simulink model "Modelo_Red_Mitigación_final"  (R2019b)
settings: Solver=VariableStepAuto  StartTime=0.0  StopTime=2.5  RelTol=1e-3
InitFcn:
  | Ts=20e-6;
undefined symbols (not defined in the file): D1, Delta, Ion, Lithium
libraries: powerlib x371, powerlib_meascontrol x286, simulink x50, simulink_extras x20, electricdrivelib x16
(part 4 of 11)

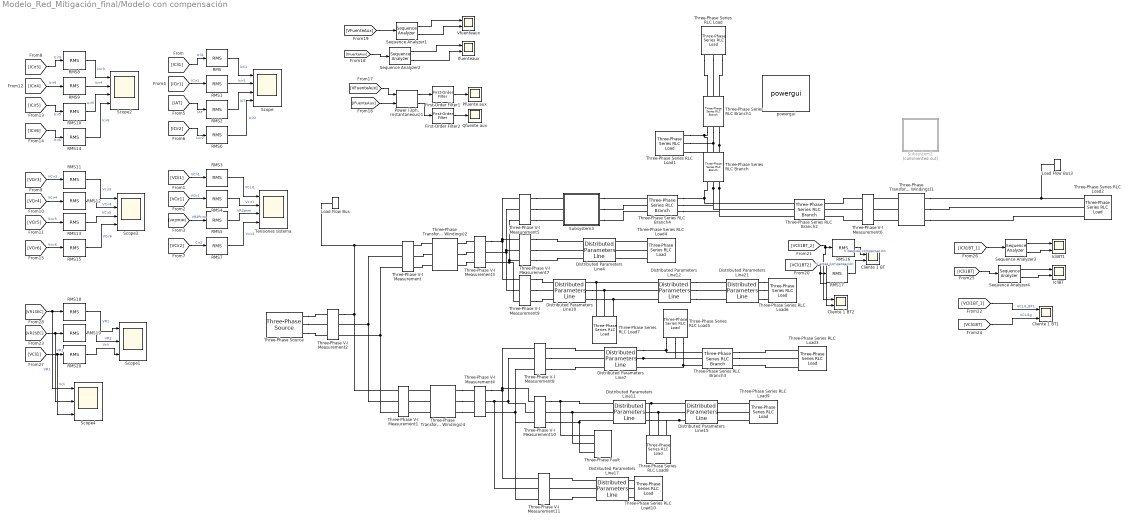
== system Modelo_Red_Mitigación_final/Modelo con compensación ==
  Cliente 1 BT : Scope  NumInputPorts=2
  Cliente 1 BT1 : Scope  NumInputPorts=3
  Cliente 1 BT2 : Scope  NumInputPorts=2
  Distributed Parameters Line10 : powerlib/Elements/Distributed Parameters Line  Phases=3  Frequency=60  Resistance=[0.213 0.639]  Inductance=[0.78e-3 2.35e-3]  Capacitance=[15e-9 15e-9]  Length=3  x1=[-2e-05 3.60953176170516e-09 32175.0070560431 -19325.0634978567;-1e-05 3.60559101207762e-09 32247.6320174573 -19203.6295402532]  x2=[-2e-05 3.3920787146718e-09 31687.8811035473 -19346.7961292865;-1e-05 3.38863307732371e-09 31760.5914564267 -19227.1984344751]  x3=[-2e-05 -6.04879747397163e-11 -137.471205101226 265.134927538772;-1e-05 -6.06175334127226e-11 -138.469760977244 264.614790455632]  x4=[-2e-05 7.88128095264096e-11 416.613031958925 -434.907199032997;-1e-05 7.89310008588255e-11 418.249629092382 -433.333518127575]  x5=1.78115131305569e-05  V1=ones(3,3)  V2=ones(3,3)  I1=ones(3,3)  I2=ones(3,3)  nHarmo=1  Measurements=None
      settings: SourceProductName=Simscape Electrical
  Distributed Parameters Line11 : powerlib/Elements/Distributed Parameters Line  Phases=3  Frequency=60  Resistance=[0.269 0.807]  Inductance=[0.85e-3 2.56e-3]  Capacitance=[15e-9 15e-9]  Length=18  x1=[-0.00012 2.25515335002305e-09 31483.0427639054 -20454.4474545806;-0.00011 2.26415722602629e-09 31559.9303096165 -20335.6141091991;-0.0001 2.27312892334362e-09 31636.3693188597 -20216.4917497281;-9e-05 2.28206831446736e-09 31712.3587052676 -20097.0820691601;-8e-05 2.29097527234899e-09 31787.8973888629 -19977.3867645708;-7e-05 2.29984967040091e-09 31862.9842960736 -19857.4075370956;-6e-05 2.30869138249829e-09 31937.6183597485 -19737.1460919048;-5e-05 2.31750028298082e-09 32011.7985191725 -19616.6041381797;-4e-05 2.32627624665453e-09 32085.5237200813 -19495.7833890884;-3e-05 2.33501914879354e-09 32158.7929146765 -19374.6855617611;-2e-05 2.34372886514188e-09 32231.6050616407 -19253.312377266;-1e-05 2.35240527191519e-09 32303.9591261522 -19131.6655605847]  x2=[-0.00012 1.94941502653526e-09 29675.6367944921 -20128.6580942059;-0.00011 1.95749754273358e-09 29751.3089897787 -20016.6408077573;-0.0001 1.9655522385589e-09 29826.5583531098 -19904.3390405358;-9e-05 1.97357899953614e-09 29901.3838150256 -19791.7543885982;-8e-05 1.98157771158727e-09 29975.7843120904 -19678.8884520216;-7e-05 1.98954826103289e-09 30049.7587869086 -19565.7428348808;-6e-05 1.99749053459384e-09 30123.3061881392 -19452.3191452254;-5e-05 2.00540441939284e-09 30196.4254705107 -19338.6189950572;-4e-05 2.01328980295607e-09 30269.1155948363 -19224.6440003069;-3e-05 2.02114657321477e-09 30341.3755280285 -19110.3957808115;-2e-05 2.02897461850684e-09 30413.2042431137 -18995.8759602911;-1e-05 2.03677382757844e-09 30484.6007192467 -18881.0861663258]  x3=[-0.00012 5.15773485528783e-12 9.28421720699589 123.310848994962;-0.00011 5.11579108823116e-12 8.81928138472589 123.344973326285;-0.0001 5.0737746144593e-12 8.35422022094588 123.377344652512;-9e-05 5.03168603111934e-12 7.88904032520442 123.407962513576;-8e-05 4.98952593638322e-12 7.42374830873751 123.436826474328;-7e-05 4.9472949294392e-12 6.95835078437463 123.463936124547;-6e-05 4.90499361048336e-12 6.49285436644475 123.489291078947;-5e-05 4.86262258071109e-12 6.02726567068236 123.512890977175;-4e-05 4.82018244230851e-12 5.5615913141334 123.534735483827;-3e-05 4.77767379844393e-12 5.09583791506126 123.554824288443;-2e-05 4.73509725325926e-12 4.63001209285268 123.573157105516;-1e-05 4.69245341186146e-12 4.16412046792371 123.589733674497]  x4=[-0.00012 5.1467508786483e-12 241.702417431134 -294.296225052516;-0.00011 5.23026920454686e-12 242.810167870273 -293.382939263731;-0.0001 5.31371319674279e-12 243.914467439464 -292.465483853974;-9e-05 5.39708166931226e-12 245.015300444167 -291.543871862318;-8e-05 5.48037343740475e-12 246.112651239108 -290.618116386908;-7e-05 5.56358731725985e-12 247.206504228504 -289.68823058478;-6e-05 5.64672212622414e-12 248.296843866281 -288.754227671669;-5e-05 5.72977668276798e-12 249.383654656301 -287.816120921824;-4e-05 5.81274980650226e-12 250.466921152576 -286.873923667818;-3e-05 5.89564031819523e-12 251.546627959491 -285.92764930036;-2e-05 5.97844703978925e-12 252.622759732024 -284.977311268103;-1e-05 6.06116879441752e-12 253.695301175959 -284.022923077453]  x5=0.000111541920370774  V1=ones(3,3)  V2=ones(3,3)  I1=ones(3,3)  I2=ones(3,3)  nHarmo=1  Measurements=None
      settings: SourceProductName=Simscape Electrical
  Distributed Parameters Line12 : powerlib/Elements/Distributed Parameters Line  Phases=3  Frequency=60  Resistance=[0.269 0.807]  Inductance=[0.85e-3 2.56e-3]  Capacitance=[15e-9 15e-9]  Length=6  x1=[-4e-05 3.40065095400314e-09 0 0;-3e-05 3.39730015910595e-09 31614.7203957361 -19466.1188633006;-2e-05 3.39390108105356e-09 31687.8811035473 -19346.7961292865;-1e-05 3.39045376815439e-09 31760.5914564267 -19227.1984344751]  x2=[-4e-05 3.45797591228592e-09 0 0;-3e-05 3.45530178649685e-09 30837.5027565935 -19380.3404703211;-2e-05 3.45257855322106e-09 30910.3456112392 -19263.9483803875;-1e-05 3.44980625116172e-09 30982.7491614535 -19147.2825071065]  x3=[-4e-05 -3.69816611276407e-12 0 0;-3e-05 -3.61783769618688e-12 -40.501984824249 176.337783353379;-2e-05 -3.53745786212792e-12 -41.1664732198401 176.183841754365;-1e-05 -3.45702775296255e-12 -41.8303765487246 176.027396192976]  x4=[-4e-05 1.96504684539837e-11 0 0;-3e-05 1.95629170007581e-11 300.866672819785 -339.753955836259;-2e-05 1.94750875151792e-11 302.145374033175 -338.617303560211;-1e-05 1.93869812454986e-11 303.419781092 -337.475838782748]  x5=3.71806401235912e-05  V1=ones(3,3)  V2=ones(3,3)  I1=ones(3,3)  I2=ones(3,3)  nHarmo=1  Measurements=None
      settings: SourceProductName=Simscape Electrical
  Distributed Parameters Line15 : powerlib/Elements/Distributed Parameters Line  Phases=3  Frequency=60  Resistance=[0.269 0.807]  Inductance=[0.85e-3 2.56e-3]  Capacitance=[15e-9 15e-9]  Length=12  x1=[-8e-05 1.98156914110105e-09 0 0;-7e-05 1.98954076159097e-09 0 0;-6e-05 1.99748410630282e-09 0 0;-5e-05 2.00539906234407e-09 30196.4254705107 -19338.6189950572;-4e-05 2.01328551722569e-09 30269.1155948363 -19224.6440003069;-3e-05 2.02114335886368e-09 30341.3755280285 -19110.3957808115;-2e-05 2.02897247558074e-09 30413.2042431137 -18995.8759602911;-1e-05 2.03677275610778e-09 30484.6007192467 -18881.0861663258]  x2=[-8e-05 1.91667238330513e-09 0 0;-7e-05 1.92456740683708e-09 0 0;-6e-05 1.93243507800613e-09 0 0;-5e-05 1.94027528499527e-09 29816.1536069817 -19273.9878791696;-4e-05 1.94808791637781e-09 29888.6027805703 -19161.4469314506;-3e-05 1.95587286111894e-09 29960.6271709548 -19048.6336571567;-2e-05 1.96363000857739e-09 30032.2257545092 -18935.5496596142;-1e-05 1.97135924850691e-09 30103.3975136591 -18822.1965459972]  x3=[-8e-05 2.70938359599311e-12 0 0;-7e-05 2.71078492729944e-12 0 0;-6e-05 2.71214773235161e-12 0 0;-5e-05 2.71347199178116e-12 86.3403246372415 -15.5892894445469;-4e-05 2.71475768676741e-12 86.3984811911008 -15.2636840808873;-3e-05 2.71600479903781e-12 86.455409831299 -14.9378617864907;-2e-05 2.71721331086812e-12 86.5111097487539 -14.611827192013;-1e-05 2.71838320508272e-12 86.5655801518465 -14.2855849311276]  x4=[-8e-05 6.06852121097726e-12 0 0;-7e-05 6.10206473358783e-12 0 0;-6e-05 6.13552153235158e-12 0 0;-5e-05 6.16889113177335e-12 161.91207626267 -146.998141908763;-4e-05 6.20217305759727e-12 162.465094324763 -146.38670462294;-3e-05 6.23536683681349e-12 163.015803398247 -145.773186858016;-2e-05 6.26847199766495e-12 163.564195656329 -145.157597333438;-1e-05 6.30148806965402e-12 164.11026330514 -144.539944798094]  x5=7.43612802471824e-05  V1=ones(3,3)  V2=ones(3,3)  I1=ones(3,3)  I2=ones(3,3)  nHarmo=1  Measurements=None
      settings: SourceProductName=Simscape Electrical
  Distributed Parameters Line17 : powerlib/Elements/Distributed Parameters Line  Phases=3  Frequency=60  Resistance=[0.213 0.639]  Inductance=[0.78e-3 2.35e-3]  Capacitance=[15e-9 15e-9]  Length=18  x1=[-0.00011 2.26415722602629e-09 31559.9303096165 -20335.6141091991;-0.0001 2.27312892334362e-09 31636.3693188597 -20216.4917497281;-9e-05 2.28206831446736e-09 31712.3587052676 -20097.0820691601;-8e-05 2.29097527234899e-09 31787.8973888629 -19977.3867645708;-7e-05 2.29984967040091e-09 31862.9842960736 -19857.4075370956;-6e-05 2.30869138249829e-09 31937.6183597485 -19737.1460919048;-5e-05 2.31750028298082e-09 32011.7985191725 -19616.6041381797;-4e-05 2.32627624665453e-09 32085.5237200813 -19495.7833890884;-3e-05 2.33501914879354e-09 32158.7929146765 -19374.6855617611;-2e-05 2.34372886514188e-09 32231.6050616407 -19253.312377266;-1e-05 2.35240527191519e-09 32303.9591261522 -19131.6655605847]  x2=[-0.00011 2.16599636455895e-09 30839.7793585705 -20381.2716559546;-0.0001 2.17462439466361e-09 30916.3956097717 -20264.8638707302;-9e-05 2.18322151854208e-09 30992.5724705577 -20148.1680769337;-8e-05 2.1917876140102e-09 31068.3088582867 -20031.1859330708;-7e-05 2.20032255932479e-09 31143.6036965769 -19913.9191017167;-6e-05 2.20882623318538e-09 31218.4559153221 -19796.3692494926;-5e-05 2.21729851473596e-09 31292.8644507065 -19678.538047042;-4e-05 2.22573928356664e-09 31366.8282452201 -19560.4271690073;-3e-05 2.23414841971541e-09 31440.3462476737 -19442.0382940054;-2e-05 2.24252580366984e-09 31513.4174132138 -19323.3731046042;-1e-05 2.25087131636876e-09 31586.0407033373 -19204.4332872989]  x3=[-0.00011 5.75160708206705e-12 65.9317893508161 -5.21472769211793;-0.0001 5.74612435792413e-12 65.9509798461658 -4.96613423438911;-9e-05 5.74055996863501e-12 65.9692330321091 -4.71747019690026;-8e-05 5.73491399328197e-12 65.9865486492278 -4.46873911371776;-7e-05 5.72918651210683e-12 66.0029264514285 -4.21994451986088;-6e-05 5.72337760650976e-12 66.0183662059466 -3.97108995125151;-5e-05 5.71748735904818e-12 66.0328676933488 -3.7221789446639;-4e-05 5.71151585343554e-12 66.0464307075371 -3.47321503767442;-3e-05 5.70546317454015e-12 66.0590550557509 -3.22420176861127;-2e-05 5.69932940838398e-12 66.0707405585703 -2.97514267650421;-1e-05 5.69311464214142e-12 66.0814870499183 -2.72604130103422]  x4=[-0.00011 4.31568373195511e-12 202.227351702517 -174.253957712798;-0.0001 4.36167015875297e-12 202.882835041406 -173.490342096467;-9e-05 4.40759459656329e-12 203.535434966127 -172.724260798352;-8e-05 4.45345639269816e-12 204.185142201791 -171.955724706166;-7e-05 4.49925489535994e-12 204.831947514619 -171.184744742506;-6e-05 4.54498945365053e-12 205.475841712076 -170.411331864706;-5e-05 4.59065941758063e-12 206.116815643 -169.635497064673;-4e-05 4.63626413807896e-12 206.754860197734 -168.857251368738;-3e-05 4.68180296700149e-12 207.389966308251 -168.076605837494;-2e-05 4.72727525714066e-12 208.022124948288 -167.293571565643;-1e-05 4.77268036223458e-12 208.651327133471 -166.508159681835]  x5=0.000106869078783341  V1=ones(3,3)  V2=ones(3,3)  I1=ones(3,3)  I2=ones(3,3)  nHarmo=1  Measurements=None
      settings: SourceProductName=Simscape Electrical
  Distributed Parameters Line21 : powerlib/Elements/Distributed Parameters Line  Phases=3  Frequency=60  Resistance=[0.269 0.807]  Inductance=[0.85e-3 2.56e-3]  Capacitance=[15e-9 15e-9]  Length=3  x1=[-2e-05 3.45441977735251e-09 30910.3456112392 -19263.9483803875;-1e-05 3.45163637093425e-09 30982.7491614535 -19147.2825071065]  x2=[-2e-05 3.12977626724445e-09 30521.2143171991 -19221.4149453172;-1e-05 3.12742225506452e-09 30593.4602857292 -19106.216361226]  x3=[-2e-05 -7.08035851296492e-11 -43.7280619986038 177.821448028224;-1e-05 -7.09955174729478e-11 -44.398120740149 177.655333890518]  x4=[-2e-05 8.23431902033655e-11 300.811121285787 -339.602032284616;-1e-05 8.25181278003377e-11 302.089250156992 -338.465590512005]  x5=1.85903200617956e-05  V1=ones(3,3)  V2=ones(3,3)  I1=ones(3,3)  I2=ones(3,3)  nHarmo=1  Measurements=None
      settings: SourceProductName=Simscape Electrical
  Distributed Parameters Line4 : powerlib/Elements/Distributed Parameters Line  Phases=3  Frequency=60  Resistance=[0.213 0.639]  Inductance=[0.78e-3 2.35e-3]  Capacitance=[15e-9 15e-9]  Length=9  x1=[-6e-05 3.62494578097809e-09 31879.9448486981 -19808.035609231;-5e-05 3.62118313403904e-09 31954.3926645073 -19687.7105752568;-4e-05 3.61736902207213e-09 32028.3863376657 -19567.1057353365;-3e-05 3.61350349928436e-09 32101.9248165591 -19446.2228035317;-2e-05 3.60958662061336e-09 32175.0070560431 -19325.0634978567;-1e-05 3.60561844172663e-09 32247.6320174573 -19203.6295402532]  x2=[-6e-05 3.32131517644419e-09 31220.7541322128 -19854.186340228;-5e-05 3.3181246812965e-09 31295.3806160466 -19736.34606287;-4e-05 3.3148870282524e-09 31369.5623232492 -19618.225288348;-3e-05 3.31160226332611e-09 31443.2981995346 -19499.8256954195;-2e-05 3.30827043320141e-09 31516.5871969527 -19381.148966805;-1e-05 3.30489158523098e-09 31589.4282739045 -19262.1967891634]  x3=[-6e-05 -2.09677278907869e-11 9.19435123996087 67.3100361697703;-5e-05 -2.10349486785391e-11 8.940533646812 67.3442196629359;-4e-05 -2.11018705131096e-11 8.6865889888901 67.3774460456733;-3e-05 -2.1168492443391e-11 8.43252087531085 67.4097148457621;-2e-05 -2.12348135225382e-11 8.17833291694453 67.4410256045912;-1e-05 -2.13008328079819e-11 7.92402872636468 67.4713778771654]  x4=[-6e-05 3.87950361892921e-11 264.77686067222 -241.746580654783;-5e-05 3.88437674883829e-11 265.686340119013 -240.746679893785;-4e-05 3.88919467315569e-11 266.592043574815 -239.743357589571;-3e-05 3.89395732340802e-11 267.493958167574 -238.736628001573;-2e-05 3.8986646319075e-11 268.392071079089 -237.726505437646;-1e-05 3.90331653175284e-11 269.286369545186 -236.713004253869]  x5=5.34345393916706e-05  V1=ones(3,3)  V2=ones(3,3)  I1=ones(3,3)  I2=ones(3,3)  nHarmo=1  Measurements=None
      settings: SourceProductName=Simscape Electrical
  Distributed Parameters Line7 : powerlib/Elements/Distributed Parameters Line  Phases=3  Frequency=60  Resistance=[0.213 0.639]  Inductance=[0.78e-3 2.35e-3]  Capacitance=[15e-9 15e-9]  Length=4.4  x1=[-3e-05 2.33501914879354e-09 0 0;-2e-05 2.34372886514188e-09 32231.6050616407 -19253.312377266;-1e-05 2.35240527191519e-09 32303.9591261522 -19131.6655605847]  x2=[-3e-05 2.3341247230935e-09 0 0;-2e-05 2.34252623298859e-09 31928.0322823421 -19306.2030460024;-1e-05 2.35089445040071e-09 32000.5878967254 -19185.7002931794]  x3=[-3e-05 1.99264250802803e-11 0 0;-2e-05 1.99128470822932e-11 2.67417656213937 49.6193899931833;-1e-05 1.98989860786719e-11 2.4870973089527 49.6291187767515]  x4=[-3e-05 -9.06267120981607e-12 0 0;-2e-05 -9.01088750737564e-12 277.339936666597 -218.990274984951;-1e-05 -8.95897574027808e-12 278.163537790781 -217.943174364175]  x5=2.61235525914834e-05  V1=ones(3,3)  V2=ones(3,3)  I1=ones(3,3)  I2=ones(3,3)  nHarmo=1  Measurements=None
      settings: SourceProductName=Simscape Electrical
  First-Order Filter1 : powerlib_meascontrol/Filters/First-Order Filter  FilterType=Lowpass  Tc=10e-3  Ts=0  Initialize=on  Vac_Init=[0, 0, 60]  Vdc_Init=0  PlotResponse=off  FreqRange="[0,  200,  1]"
      settings: SourceProductName=Simscape Electrical
  First-Order Filter2 : powerlib_meascontrol/Filters/First-Order Filter  FilterType=Lowpass  Tc=10e-3  Ts=0  Initialize=on  Vac_Init=[0, 0, 60]  Vdc_Init=0  PlotResponse=off  FreqRange="[0,  200,  1]"
      settings: SourceProductName=Simscape Electrical
  IcliBT : Scope  NumInputPorts=2
  IcliBT1 : Scope  NumInputPorts=2
  Ifuenteaux : Scope  NumInputPorts=2
  Load Flow Bus : powerlib/Measurements/Load Flow Bus  LConnTagsString=a  Phases=single  Connectors=on one side  ID=BUS_1  Vbase=115e3  Vref=1.05  Vangle=0  VLF=1  VLFb=1  VLFc=1  angleLF=0  angleLFb=0  angleLFc=0
      settings: SourceProductName=Simscape Electrical
  Load Flow Bus3 : powerlib/Measurements/Load Flow Bus  LConnTagsString=a  Phases=single  Connectors=on one side  ID=BUS_4  Vbase=440  Vref=1  Vangle=0  VLF=0.9785  VLFb=1  VLFc=1  angleLF=28.33  angleLFb=0  angleLFc=0
      settings: SourceProductName=Simscape Electrical
  "Pfuente aux " : Scope
  "Power (3ph, Instantaneous)1" : powerlib_meascontrol/Measurements/Power (3ph, Instantaneous)
      settings: SourceProductName=Simscape Electrical
  Qfuente aux : Scope
  RMS{,1..20} (21 alike) : powerlib_meascontrol/Measurements/RMS  TrueRMS=on  Freq=60  RMSInit=120  Ts=0
      settings: SourceProductName=Simscape Electrical
  Scope : Scope  NumInputPorts=4
  Scope1 : Scope  NumInputPorts=3
  Scope2 : Scope  NumInputPorts=4
  Scope3 : Scope  NumInputPorts=4
  Scope4 : Scope  NumInputPorts=3
  Sequence Analyzer{1..4} (4 alike) : powerlib_meascontrol/Measurements/Sequence Analyzer  Freq=60  n=1  seq=Positive Negative Zero  InInit=[1, 0]  Ts=0
      settings: SourceProductName=Simscape Electrical  SourceProductBaseCode=PS
  Subsystem2 : Subsystem  Commented=on
  Subsystem3 : Subsystem
  Tensiones sistema : Scope  NumInputPorts=4
  Three-Phase Series RLC Branch : powerlib/Elements/Three-Phase Series RLC Branch  LConnTagsString=A|B|C  RConnTagsString=A|B|C  BranchType=RL  Resistance=0.213  Inductance=0.78e-3  Capacitance=1e-6  Measurements=None
      settings: SourceProductName=Simscape Electrical
  Three-Phase Series RLC Branch1 : powerlib/Elements/Three-Phase Series RLC Branch  LConnTagsString=A|B|C  RConnTagsString=A|B|C  BranchType=RL  Resistance=0.213  Inductance=0.78e-3  Capacitance=1e-6  Measurements=None
      settings: SourceProductName=Simscape Electrical
  Three-Phase Series RLC Branch2 : powerlib/Elements/Three-Phase Series RLC Branch  LConnTagsString=A|B|C  RConnTagsString=A|B|C  BranchType=RL  Resistance=0.213*1.7  Inductance=0.78e-3*1.7  Capacitance=1e-6  Measurements=None
      settings: SourceProductName=Simscape Electrical
  Three-Phase Series RLC Branch3 : powerlib/Elements/Three-Phase Series RLC Branch  LConnTagsString=A|B|C  RConnTagsString=A|B|C  BranchType=RL  Resistance=0.213*2.2  Inductance=0.78e-3*2.2  Capacitance=1e-6  Measurements=None
      settings: SourceProductName=Simscape Electrical
  Three-Phase Series RLC Branch4 : powerlib/Elements/Three-Phase Series RLC Branch  LConnTagsString=A|B|C  RConnTagsString=A|B|C  BranchType=RL  Resistance=0.213*7  Inductance=0.78e-3*7  Capacitance=1e-6  Measurements=None
      settings: SourceProductName=Simscape Electrical
  Three-Phase Series RLC Load : powerlib/Elements/Three-Phase Series RLC Load  LConnTagsString=A|B|C  Configuration=Y (grounded)  NominalVoltage=34.5e3  Vabc=[1e3 1e3 1e3]  Vabcp=[1e3 1e3 1e3]  NominalFrequency=60  UnbalancedPower=off  ActivePower=0.5e6  InductivePower=0.1e6  CapacitivePower=0  Pabc=[10e3 9e3 11e3]  QLabc=[100 90 110]  QCabc=[100 90 110]  Pabcp=[10e3 9e3 11e3]  QLabcp=[100 90 110]  QCabcp=[100 90 110]  Measurements=None  LoadType=constant Z
      settings: SourceProductName=Simscape Electrical
  Three-Phase Series RLC Load1 : powerlib/Elements/Three-Phase Series RLC Load  LConnTagsString=A|B|C  Configuration=Y (grounded)  NominalVoltage=34.5e3  Vabc=[1e3 1e3 1e3]  Vabcp=[1e3 1e3 1e3]  NominalFrequency=60  UnbalancedPower=off  ActivePower=2.5e6  InductivePower=1e6  CapacitivePower=0  Pabc=[10e3 9e3 11e3]  QLabc=[100 90 110]  QCabc=[100 90 110]  Pabcp=[10e3 9e3 11e3]  QLabcp=[100 90 110]  QCabcp=[100 90 110]  Measurements=None  LoadType=constant Z
      settings: SourceProductName=Simscape Electrical
  Three-Phase Series RLC Load10 : powerlib/Elements/Three-Phase Series RLC Load  LConnTagsString=A|B|C  Configuration=Y (grounded)  NominalVoltage=34.5e3  Vabc=[1e3 1e3 1e3]  Vabcp=[1e3 1e3 1e3]  NominalFrequency=60  UnbalancedPower=off  ActivePower=3.4e6  InductivePower=1.1e6  CapacitivePower=0  Pabc=[10e3 9e3 11e3]  QLabc=[100 90 110]  QCabc=[100 90 110]  Pabcp=[10e3 9e3 11e3]  QLabcp=[100 90 110]  QCabcp=[100 90 110]  Measurements=None  LoadType=constant Z
      settings: SourceProductName=Simscape Electrical
  Three-Phase Series RLC Load2 : powerlib/Elements/Three-Phase Series RLC Load  LConnTagsString=A|B|C  Configuration=Y (grounded)  NominalVoltage=440  Vabc=[1e3 1e3 1e3]  Vabcp=[1e3 1e3 1e3]  NominalFrequency=60  UnbalancedPower=off  ActivePower=6.5e6  InductivePower=3e6  CapacitivePower=0  Pabc=[10e3 9e3 11e3]  QLabc=[100 90 110]  QCabc=[100 90 110]  Pabcp=[10e3 9e3 11e3]  QLabcp=[100 90 110]  QCabcp=[100 90 110]  Measurements=None  LoadType=constant Z
      settings: SourceProductName=Simscape Electrical
  Three-Phase Series RLC Load3 : powerlib/Elements/Three-Phase Series RLC Load  LConnTagsString=A|B|C  Configuration=Y (grounded)  NominalVoltage=34.5e3  Vabc=[1e3 1e3 1e3]  Vabcp=[1e3 1e3 1e3]  NominalFrequency=60  UnbalancedPower=off  ActivePower=3e6  InductivePower=0.7e6  CapacitivePower=0  Pabc=[10e3 9e3 11e3]  QLabc=[100 90 110]  QCabc=[100 90 110]  Pabcp=[10e3 9e3 11e3]  QLabcp=[100 90 110]  QCabcp=[100 90 110]  Measurements=None  LoadType=constant Z
      settings: SourceProductName=Simscape Electrical
  Three-Phase Series RLC Load4 : powerlib/Elements/Three-Phase Series RLC Load  LConnTagsString=A|B|C  Configuration=Y (grounded)  NominalVoltage=34.5e3  Vabc=[1e3 1e3 1e3]  Vabcp=[1e3 1e3 1e3]  NominalFrequency=60  UnbalancedPower=off  ActivePower=6.2e6  InductivePower=2e6  CapacitivePower=0  Pabc=[10e3 9e3 11e3]  QLabc=[100 90 110]  QCabc=[100 90 110]  Pabcp=[10e3 9e3 11e3]  QLabcp=[100 90 110]  QCabcp=[100 90 110]  Measurements=None  LoadType=constant Z
      settings: SourceProductName=Simscape Electrical
  Three-Phase Series RLC Load5 : powerlib/Elements/Three-Phase Series RLC Load  LConnTagsString=A|B|C  Configuration=Y (grounded)  NominalVoltage=34.5e3  Vabc=[1e3 1e3 1e3]  Vabcp=[1e3 1e3 1e3]  NominalFrequency=60  UnbalancedPower=off  ActivePower=3e6  InductivePower=0.7e6  CapacitivePower=0  Pabc=[10e3 9e3 11e3]  QLabc=[100 90 110]  QCabc=[100 90 110]  Pabcp=[10e3 9e3 11e3]  QLabcp=[100 90 110]  QCabcp=[100 90 110]  Measurements=None  LoadType=constant Z
      settings: SourceProductName=Simscape Electrical
  Three-Phase Series RLC Load6 : powerlib/Elements/Three-Phase Series RLC Load  LConnTagsString=A|B|C  Configuration=Y (grounded)  NominalVoltage=34.5e3  Vabc=[1e3 1e3 1e3]  Vabcp=[1e3 1e3 1e3]  NominalFrequency=60  UnbalancedPower=off  ActivePower=9.4e6  InductivePower=4.2e6  CapacitivePower=0  Pabc=[10e3 9e3 11e3]  QLabc=[100 90 110]  QCabc=[100 90 110]  Pabcp=[10e3 9e3 11e3]  QLabcp=[100 90 110]  QCabcp=[100 90 110]  Measurements=None  LoadType=constant Z
      settings: SourceProductName=Simscape Electrical
  Three-Phase Series RLC Load7 : powerlib/Elements/Three-Phase Series RLC Load  LConnTagsString=A|B|C  Configuration=Y (grounded)  NominalVoltage=34.5e3  Vabc=[1e3 1e3 1e3]  Vabcp=[1e3 1e3 1e3]  NominalFrequency=60  UnbalancedPower=off  ActivePower=4.4e6  InductivePower=0.8e6  CapacitivePower=0  Pabc=[10e3 9e3 11e3]  QLabc=[100 90 110]  QCabc=[100 90 110]  Pabcp=[10e3 9e3 11e3]  QLabcp=[100 90 110]  QCabcp=[100 90 110]  Measurements=None  LoadType=constant Z
      settings: SourceProductName=Simscape Electrical
  Three-Phase Series RLC Load8 : powerlib/Elements/Three-Phase Series RLC Load  LConnTagsString=A|B|C  Configuration=Y (grounded)  NominalVoltage=34.5e3  Vabc=[1e3 1e3 1e3]  Vabcp=[1e3 1e3 1e3]  NominalFrequency=60  UnbalancedPower=off  ActivePower=5e6  InductivePower=2.5e6  CapacitivePower=0  Pabc=[10e3 9e3 11e3]  QLabc=[100 90 110]  QCabc=[100 90 110]  Pabcp=[10e3 9e3 11e3]  QLabcp=[100 90 110]  QCabcp=[100 90 110]  Measurements=None  LoadType=constant Z
      settings: SourceProductName=Simscape Electrical
  Three-Phase Series RLC Load9 : powerlib/Elements/Three-Phase Series RLC Load  LConnTagsString=A|B|C  Configuration=Y (grounded)  NominalVoltage=34.5e3  Vabc=[1e3 1e3 1e3]  Vabcp=[1e3 1e3 1e3]  NominalFrequency=60  UnbalancedPower=off  ActivePower=2.3e6  InductivePower=1.2e6  CapacitivePower=0  Pabc=[10e3 9e3 11e3]  QLabc=[100 90 110]  QCabc=[100 90 110]  Pabcp=[10e3 9e3 11e3]  QLabcp=[100 90 110]  QCabcp=[100 90 110]  Measurements=None  LoadType=constant Z
      settings: SourceProductName=Simscape Electrical
  Three-Phase V-I Measurement : powerlib/Measurements/Three-Phase V-I Measurement  VoltageMeasurement=phase-to-ground  SetLabelV=on  LabelV=VR2PRIM  Vpu=off  VpuLL=off  CurrentMeasurement=yes  SetLabelI=on  LabelI=IR2PRIM  Ipu=off  Pbase=100e6  Vbase=500e3  OutputType=Complex  PhasorSimulation=off  PSBequivalent=0
      settings: SourceProductName=Simscape Electrical
  Three-Phase V-I Measurement1 : powerlib/Measurements/Three-Phase V-I Measurement  VoltageMeasurement=phase-to-ground  SetLabelV=on  LabelV=VR1PRIM  Vpu=off  VpuLL=off  CurrentMeasurement=yes  SetLabelI=on  LabelI=IR1PRIM  Ipu=off  Pbase=100e6  Vbase=500e3  OutputType=Complex  PhasorSimulation=off  PSBequivalent=0
      settings: SourceProductName=Simscape Electrical
  Three-Phase V-I Measurement10 : powerlib/Measurements/Three-Phase V-I Measurement  VoltageMeasurement=phase-to-ground  SetLabelV=on  LabelV=VCir5  Vpu=off  VpuLL=off  CurrentMeasurement=yes  SetLabelI=on  LabelI=ICir5  Ipu=off  Pbase=100e6  Vbase=500e3  OutputType=Complex  PhasorSimulation=off  PSBequivalent=0
      settings: SourceProductName=Simscape Electrical
  Three-Phase V-I Measurement11 : powerlib/Measurements/Three-Phase V-I Measurement  VoltageMeasurement=phase-to-ground  SetLabelV=on  LabelV=VCir6  Vpu=off  VpuLL=off  CurrentMeasurement=yes  SetLabelI=on  LabelI=ICir6  Ipu=off  Pbase=100e6  Vbase=500e3  OutputType=Complex  PhasorSimulation=off  PSBequivalent=0
      settings: SourceProductName=Simscape Electrical
  Three-Phase V-I Measurement2 : powerlib/Measurements/Three-Phase V-I Measurement  VoltageMeasurement=phase-to-ground  SetLabelV=on  LabelV=VAT  Vpu=off  VpuLL=off  CurrentMeasurement=yes  SetLabelI=on  LabelI=IAT  Ipu=off  Pbase=100e6  Vbase=500e3  OutputType=Complex  PhasorSimulation=off  PSBequivalent=0
      settings: SourceProductName=Simscape Electrical
  Three-Phase V-I Measurement3 : powerlib/Measurements/Three-Phase V-I Measurement  VoltageMeasurement=phase-to-ground  SetLabelV=on  LabelV=VR2SEC  Vpu=off  VpuLL=off  CurrentMeasurement=yes  SetLabelI=on  LabelI=IR2SEC  Ipu=off  Pbase=100e6  Vbase=500e3  OutputType=Complex  PhasorSimulation=off  PSBequivalent=0
      settings: SourceProductName=Simscape Electrical
  Three-Phase V-I Measurement4 : powerlib/Measurements/Three-Phase V-I Measurement  VoltageMeasurement=phase-to-ground  SetLabelV=on  LabelV=VR1SEC  Vpu=off  VpuLL=off  CurrentMeasurement=yes  SetLabelI=on  LabelI=IR1SEC  Ipu=off  Pbase=100e6  Vbase=500e3  OutputType=Complex  PhasorSimulation=off  PSBequivalent=0
      settings: SourceProductName=Simscape Electrical
  Three-Phase V-I Measurement5 : powerlib/Measurements/Three-Phase V-I Measurement  VoltageMeasurement=phase-to-ground  SetLabelV=on  LabelV=VCir1  Vpu=off  VpuLL=off  CurrentMeasurement=yes  SetLabelI=on  LabelI=ICir1  Ipu=off  Pbase=100e6  Vbase=500e3  OutputType=Complex  PhasorSimulation=off  PSBequivalent=0
      settings: SourceProductName=Simscape Electrical
  Three-Phase V-I Measurement6 : powerlib/Measurements/Three-Phase V-I Measurement  VoltageMeasurement=phase-to-ground  SetLabelV=on  LabelV=VCli1  Vpu=off  VpuLL=off  CurrentMeasurement=yes  SetLabelI=on  LabelI=ICli1  Ipu=off  Pbase=100e6  Vbase=500e3  OutputType=Complex  PhasorSimulation=off  PSBequivalent=0
      settings: SourceProductName=Simscape Electrical
  Three-Phase V-I Measurement7 : powerlib/Measurements/Three-Phase V-I Measurement  VoltageMeasurement=phase-to-ground  SetLabelV=on  LabelV=VCir2  Vpu=off  VpuLL=off  CurrentMeasurement=yes  SetLabelI=on  LabelI=ICir2  Ipu=off  Pbase=100e6  Vbase=500e3  OutputType=Complex  PhasorSimulation=off  PSBequivalent=0
      settings: SourceProductName=Simscape Electrical
  Three-Phase V-I Measurement8 : powerlib/Measurements/Three-Phase V-I Measurement  VoltageMeasurement=phase-to-ground  SetLabelV=on  LabelV=VCir4  Vpu=off  VpuLL=off  CurrentMeasurement=yes  SetLabelI=on  LabelI=ICir4  Ipu=off  Pbase=100e6  Vbase=500e3  OutputType=Complex  PhasorSimulation=off  PSBequivalent=0
      settings: SourceProductName=Simscape Electrical
  Three-Phase V-I Measurement9 : powerlib/Measurements/Three-Phase V-I Measurement  VoltageMeasurement=phase-to-ground  SetLabelV=on  LabelV=VCir3  Vpu=off  VpuLL=off  CurrentMeasurement=yes  SetLabelI=on  LabelI=ICir3  Ipu=off  Pbase=100e6  Vbase=500e3  OutputType=Complex  PhasorSimulation=off  PSBequivalent=0
      settings: SourceProductName=Simscape Electrical
  Three-Phase Fault : powerlib/Elements/Three-Phase Fault  InitialStates=0  FaultA=on  FaultB=on  FaultC=on  GroundFault=off  SwitchTimes=[0.1,0.9]  External=off  SwitchStatus=NaN  FaultResistance=0.3  GroundResistance=0.01  SnubberResistance=1e6  SnubberCapacitance=inf  Measurements=None
      settings: SourceProductName=Simscape Electrical
  Three-Phase Source : powerlib/Electrical Sources/Three-Phase Source  InternalConnection=Yg  VoltagePhases=off  Voltage=(115000)*1.39942  PhaseAngle=16.7311  Voltage_phases=[25e3 25e3 25e3]/sqrt(3)  PhaseAngles_phases=[0 -120 +120]  Frequency=60  NonIdealSource=on  SpecifyImpedance=on  Resistance=0.8929  Inductance=16.58e-3  ShortCircuitLevel=100e6  BaseVoltage=115e3  XRratio=5.946  BusType=swing  Pref=10e3  Qref=0  Prefabc=[10e3, 10e3, 10e3]  Qrefabc=[0, 0, 0]  Qmin=-inf  Qmax=inf
      settings: SourceProductName=Simscape Electrical
  Three-Phase Transformer Inductance Matrix Type (Two Windings)1 : powerlib/Elements/Three-Phase Transformer Inductance Matrix Type (Two Windings)  CoreType=Three-limb or five-limb core  Winding1Connection=Yg  Winding2Connection=Yg  AutoTransformer=off  Measurements=None  NominalPower=[10e6, 60]  VLLnom=[34.5e3, 440]  WindingResistances=[0.01, 0.01]  NoLoadIexcPos=2  NoLoadPlossPos=1000  ShortCircuitReactancePos=0.06  ShortCircuitReactancePosAuto=0.06  NoLoadIexcZero=100  NoLoadPlossZero=500000  ShortCircuitReactanceZero=0.03  ShortCircuitReactanceZeroAuto=0.03
      settings: SourceProductName=Simscape Electrical  SourceProductBaseCode=PS
  Three-Phase Transformer Inductance Matrix Type (Two Windings)2 : powerlib/Elements/Three-Phase Transformer Inductance Matrix Type (Two Windings)  CoreType=Three single-phase cores  Winding1Connection=Delta (D1)  Winding2Connection=Y  AutoTransformer=off  Measurements=None  NominalPower=[40e6, 60]  VLLnom=[115e3, 34.5e3]  WindingResistances=[0.006, 0.006]  NoLoadIexcPos=2  NoLoadPlossPos=16600  ShortCircuitReactancePos=0.1056  ShortCircuitReactancePosAuto=0.06  NoLoadIexcZero=100  NoLoadPlossZero=500000  ShortCircuitReactanceZero=0.1056  ShortCircuitReactanceZeroAuto=0.03
      settings: SourceProductName=Simscape Electrical  SourceProductBaseCode=PS
  Three-Phase Transformer Inductance Matrix Type (Two Windings)4 : powerlib/Elements/Three-Phase Transformer Inductance Matrix Type (Two Windings)  CoreType=Three single-phase cores  Winding1Connection=Delta (D1)  Winding2Connection=Y  AutoTransformer=off  Measurements=None  NominalPower=[30e6, 60]  VLLnom=[115e3, 34.5e3]  WindingResistances=[0.006, 0.006]  NoLoadIexcPos=2  NoLoadPlossPos=14300  ShortCircuitReactancePos=0.0912  ShortCircuitReactancePosAuto=0.06  NoLoadIexcZero=100  NoLoadPlossZero=500000  ShortCircuitReactanceZero=0.0912  ShortCircuitReactanceZeroAuto=0.03
      settings: SourceProductName=Simscape Electrical  SourceProductBaseCode=PS
  Vfuenteaux : Scope  NumInputPorts=2
  powergui : powerlib/powergui  Priority=1  SimulationMode=Discrete  SampleTime=10e-6  frequency=60  Iterations=50  frequencyindice=0  Pbase=100e6  ErrMax=0.0001  UnitsV=kV  UnitsW=MW  buscounter=0  FunctionMessages=off  echomessages=off  EnableUseOfTLC=off  CurrentSourceSwitches=off  DisableSnubberDevices=off  DisableRonSwitches=off  DisableVfSwitches=off  DisplayEquations=off  AutomaticDiscreteSolvers=off  SolverType=Tustin/Backward Euler (TBE)  Interpol=off  ExternalGateDelay=off  methode=off  Ts=100  x0status=blocks  SPID=on  SwTol=0  HookPort=off  NonlinearTolerance=1e-4  nMaxIteration=100  ContinueOnMaxIteration=off  RestoreLinks=warning  ResistiveCurrentMeasurement=off  Frange=[0:2:500]  Ylog=off  Xlog=on  ShowGrid=off  save=off  variable=ZData  structure=0  ZoomFFT=off  StartTime=0.0  cycles=1  DisplayStyle=1  fundamental=60  FreqAxis=off  MaxFrequency=1000  frequencyindicesteady=1  RmsSteady=1  display=off
      settings: SourceProductName=Simscape Electrical
  wires:
  RMS1/1 -> Scope/2  "Icir1"
  Sequence Analyzer4/2 -> IcliBT/2
  RMS5/1 -> Tensiones sistema/3  "VR2prim"
  [VCli1] -> RMS3/1  "VCli1"
  "Power (3ph, Instantaneous)1"/2 -> First-Order Filter2/1
  RMS13/1 -> Scope3/3  "VCir5"
  [ICir5] -> RMS10/1  "Icir5"
  Sequence Analyzer1/2 -> Vfuenteaux/2
  [ICir2] -> RMS6/1  "Icir2"
  RMS7/1 -> Tensiones sistema/4  "Vcir2"
  Sequence Analyzer3/1 -> IcliBT1/1
  Sequence Analyzer4/1 -> IcliBT/1
  RMS9/1 -> Scope2/2  "Icir4"
  [VCir3] -> RMS11/1  "VCir3"
  [VFuenteAux] -> Sequence Analyzer1/1
  [VCir5] -> RMS13/1  "Vcir5"
  [VCli1BT2] -> Cliente 1 BT2/2, RMS17/1
  [ICir1] -> RMS1/1  "ICir1"
  [VCir6] -> RMS15/1  "Vcir6"
  [ICli1BT] -> Sequence Analyzer4/1
  First-Order Filter1/1 -> "Pfuente aux "/1
  RMS3/1 -> Tensiones sistema/1  "VCLI1"
  [VCli1BT] -> Cliente 1 BT1/3  "VCLI1g"
  Sequence Analyzer3/2 -> IcliBT1/2
  Sequence Analyzer2/1 -> Ifuenteaux/1
  [VCli1BT_1] -> Cliente 1 BT1/1  "VCLI1_BT1"
  RMS17/1 -> Cliente 1 BT/2  "V antes compensación"
  RMS16/1 -> Cliente 1 BT/1  "V después compensación"
  [VCir2] -> RMS7/1  "Cir2"
  [ICli1BT_1] -> Sequence Analyzer3/1
  RMS14/1 -> Scope2/4  "Icir6"
  First-Order Filter2/1 -> Qfuente aux/1
  RMS6/1 -> Scope/4  "Icir2"
  RMS/1 -> Scope/1  "Icli1"
  [ICli1] -> RMS/1  "Icli1"
  [VCir1] -> RMS4/1  "VCir1"
  RMS4/1 -> Tensiones sistema/2  "Vcir1"
  [VR2PRIM] -> RMS5/1  "VR2Prim"
  [ICir6] -> RMS14/1  "Icir6"
  [IAT] -> RMS2/1  "IAT"
  RMS2/1 -> Scope/3  "IAT"
  RMS15/1 -> Scope3/4  "VCir6"
  [ICir3] -> RMS8/1  "Icir3"
  [VCir4] -> RMS12/1  "VCir4"
  [ICir4] -> RMS9/1  "Icir4"
  [VFuenteAux] -> "Power (3ph, Instantaneous)1"/1
  RMS12/1 -> Scope3/2  "VCir4"
  RMS10/1 -> Scope2/3  "Icir5"
  [IFuenteAux] -> "Power (3ph, Instantaneous)1"/2
  RMS11/1 -> Scope3/1  "Vcir3"
  "Power (3ph, Instantaneous)1"/1 -> First-Order Filter1/1
  RMS8/1 -> Scope2/1  "Icir3"
  [IFuenteAux] -> Sequence Analyzer2/1
  Sequence Analyzer2/2 -> Ifuenteaux/2
  Sequence Analyzer1/1 -> Vfuenteaux/1
  [VCli1BT_2] -> Cliente 1 BT2/1, RMS16/1
  [VR1SEC] -> Scope4/1, RMS18/1  "VR1"
  [VR2SEC] -> Scope4/2, RMS19/1  "VR2"
  RMS20/1 -> Scope1/3  "Vcli"
  RMS18/1 -> Scope1/1  "VR1"
  RMS19/1 -> Scope1/2  "VR2"
  [VCli1] -> Scope4/3, RMS20/1  "Vcli"
  connections:
  Three-Phase Series RLC Load9/LConn3 -- Distributed Parameters Line15/RConn3
  Three-Phase Transformer Inductance Matrix Type (Two Windings)1/RConn2 -- Three-Phase Series RLC Load2/LConn2
  Three-Phase V-I Measurement10/RConn3 -- Three-Phase Fault/LConn3 -- Distributed Parameters Line11/LConn3
  Three-Phase Transformer Inductance Matrix Type (Two Windings)2/RConn1 -- Three-Phase V-I Measurement3/LConn1
  Three-Phase V-I Measurement5/RConn3 -- Subsystem3/LConn3
  Distributed Parameters Line15/LConn3 -- Distributed Parameters Line11/RConn3 -- Three-Phase Series RLC Load8/LConn3
  Three-Phase V-I Measurement5/LConn2 -- Three-Phase V-I Measurement3/RConn2 -- Three-Phase V-I Measurement9/LConn2 -- Three-Phase V-I Measurement7/LConn2
  Distributed Parameters Line10/RConn2 -- Distributed Parameters Line12/LConn2 -- Three-Phase Series RLC Load7/LConn2
  Three-Phase Source/RConn1 -- Three-Phase V-I Measurement2/LConn1
  Subsystem3/RConn3 -- Three-Phase Series RLC Branch4/LConn3
  Three-Phase V-I Measurement6/LConn2 -- Three-Phase Series RLC Branch2/RConn2
  Three-Phase Series RLC Branch3/RConn2 -- Three-Phase Series RLC Load3/LConn2
  Three-Phase Transformer Inductance Matrix Type (Two Windings)1/RConn3 -- Three-Phase Series RLC Load2/LConn3
  Three-Phase V-I Measurement/LConn2 -- Three-Phase V-I Measurement1/LConn2 -- Three-Phase V-I Measurement2/RConn2
  Three-Phase Series RLC Branch/LConn3 -- Three-Phase Series RLC Branch2/LConn3 -- Three-Phase Series RLC Branch4/RConn3
  Distributed Parameters Line7/RConn1 -- Three-Phase Series RLC Branch3/LConn1 -- Three-Phase Series RLC Load5/LConn1
  Subsystem3/RConn2 -- Three-Phase Series RLC Branch4/LConn2
  Three-Phase V-I Measurement5/RConn1 -- Subsystem3/LConn1
  Distributed Parameters Line17/LConn1 -- Three-Phase V-I Measurement11/RConn1
  Three-Phase Transformer Inductance Matrix Type (Two Windings)4/RConn1 -- Three-Phase V-I Measurement4/LConn1
  Three-Phase V-I Measurement8/RConn3 -- Distributed Parameters Line7/LConn3
  Three-Phase Series RLC Load8/LConn2 -- Distributed Parameters Line11/RConn2 -- Distributed Parameters Line15/LConn2
  Three-Phase V-I Measurement9/RConn3 -- Distributed Parameters Line10/LConn3
  Three-Phase V-I Measurement3/RConn1 -- Three-Phase V-I Measurement9/LConn1 -- Three-Phase V-I Measurement7/LConn1 -- Three-Phase V-I Measurement5/LConn1
  Three-Phase Series RLC Branch3/RConn1 -- Three-Phase Series RLC Load3/LConn1
  Load Flow Bus3/LConn1 -- Three-Phase Transformer Inductance Matrix Type (Two Windings)1/RConn1 -- Three-Phase Series RLC Load2/LConn1
  Three-Phase Series RLC Branch3/RConn3 -- Three-Phase Series RLC Load3/LConn3
  Three-Phase Transformer Inductance Matrix Type (Two Windings)4/LConn1 -- Three-Phase V-I Measurement1/RConn1
  Three-Phase V-I Measurement5/RConn2 -- Subsystem3/LConn2
  Three-Phase V-I Measurement5/LConn3 -- Three-Phase V-I Measurement7/LConn3 -- Three-Phase V-I Measurement9/LConn3 -- Three-Phase V-I Measurement3/RConn3
  Subsystem3/RConn1 -- Three-Phase Series RLC Branch4/LConn1
  Three-Phase Transformer Inductance Matrix Type (Two Windings)4/RConn2 -- Three-Phase V-I Measurement4/LConn2
  Three-Phase Series RLC Branch4/RConn1 -- Three-Phase Series RLC Branch/LConn1 -- Three-Phase Series RLC Branch2/LConn1
  Three-Phase Transformer Inductance Matrix Type (Two Windings)4/RConn3 -- Three-Phase V-I Measurement4/LConn3
  Three-Phase V-I Measurement3/LConn3 -- Three-Phase Transformer Inductance Matrix Type (Two Windings)2/RConn3
  Distributed Parameters Line12/RConn3 -- Distributed Parameters Line21/LConn3
  Three-Phase Series RLC Load1/LConn1 -- Three-Phase Series RLC Branch1/LConn1 -- Three-Phase Series RLC Branch/RConn1
  Distributed Parameters Line10/RConn3 -- Distributed Parameters Line12/LConn3 -- Three-Phase Series RLC Load7/LConn3
  Three-Phase V-I Measurement2/RConn1 -- Load Flow Bus/LConn1 -- Three-Phase V-I Measurement/LConn1 -- Three-Phase V-I Measurement1/LConn1
  Three-Phase Source/RConn2 -- Three-Phase V-I Measurement2/LConn2
  Three-Phase Source/RConn3 -- Three-Phase V-I Measurement2/LConn3
  Three-Phase V-I Measurement4/RConn1 -- Three-Phase V-I Measurement11/LConn1 -- Three-Phase V-I Measurement10/LConn1 -- Three-Phase V-I Measurement8/LConn1
  Distributed Parameters Line21/RConn2 -- Three-Phase Series RLC Load6/LConn2
  Three-Phase Transformer Inductance Matrix Type (Two Windings)2/RConn2 -- Three-Phase V-I Measurement3/LConn2
  Three-Phase Transformer Inductance Matrix Type (Two Windings)4/LConn2 -- Three-Phase V-I Measurement1/RConn2
  Three-Phase Series RLC Load9/LConn2 -- Distributed Parameters Line15/RConn2
  Three-Phase Transformer Inductance Matrix Type (Two Windings)4/LConn3 -- Three-Phase V-I Measurement1/RConn3
  Three-Phase Series RLC Branch/LConn2 -- Three-Phase Series RLC Branch4/RConn2 -- Three-Phase Series RLC Branch2/LConn2
  Three-Phase Series RLC Load1/LConn2 -- Three-Phase Series RLC Branch1/LConn2 -- Three-Phase Series RLC Branch/RConn2
  Three-Phase Series RLC Load1/LConn3 -- Three-Phase Series RLC Branch1/LConn3 -- Three-Phase Series RLC Branch/RConn3
  Three-Phase V-I Measurement6/LConn1 -- Three-Phase Series RLC Branch2/RConn1
  Three-Phase Transformer Inductance Matrix Type (Two Windings)1/LConn2 -- Three-Phase V-I Measurement6/RConn2
  Three-Phase Series RLC Load/LConn1 -- Three-Phase Series RLC Branch1/RConn1
  Three-Phase Transformer Inductance Matrix Type (Two Windings)1/LConn1 -- Three-Phase V-I Measurement6/RConn1
  Three-Phase V-I Measurement6/LConn3 -- Three-Phase Series RLC Branch2/RConn3
  Three-Phase Series RLC Load8/LConn1 -- Distributed Parameters Line11/RConn1 -- Distributed Parameters Line15/LConn1
  Three-Phase V-I Measurement7/RConn1 -- Distributed Parameters Line4/LConn1
  Three-Phase V-I Measurement/LConn3 -- Three-Phase V-I Measurement1/LConn3 -- Three-Phase V-I Measurement2/RConn3
  Three-Phase V-I Measurement7/RConn2 -- Distributed Parameters Line4/LConn2
  Distributed Parameters Line7/RConn2 -- Three-Phase Series RLC Branch3/LConn2 -- Three-Phase Series RLC Load5/LConn2
  Three-Phase V-I Measurement8/RConn1 -- Distributed Parameters Line7/LConn1
  Three-Phase Series RLC Load/LConn2 -- Three-Phase Series RLC Branch1/RConn2
  Three-Phase V-I Measurement9/RConn1 -- Distributed Parameters Line10/LConn1
  Distributed Parameters Line17/LConn3 -- Three-Phase V-I Measurement11/RConn3
  Distributed Parameters Line17/RConn3 -- Three-Phase Series RLC Load10/LConn3
  Three-Phase V-I Measurement8/LConn3 -- Three-Phase V-I Measurement10/LConn3 -- Three-Phase V-I Measurement11/LConn3 -- Three-Phase V-I Measurement4/RConn3
  Three-Phase V-I Measurement9/RConn2 -- Distributed Parameters Line10/LConn2
  Distributed Parameters Line17/LConn2 -- Three-Phase V-I Measurement11/RConn2
  Three-Phase V-I Measurement8/RConn2 -- Distributed Parameters Line7/LConn2
  Three-Phase V-I Measurement10/RConn1 -- Three-Phase Fault/LConn1 -- Distributed Parameters Line11/LConn1
  Distributed Parameters Line11/LConn2 -- Three-Phase Fault/LConn2 -- Three-Phase V-I Measurement10/RConn2
  Distributed Parameters Line12/LConn1 -- Distributed Parameters Line10/RConn1 -- Three-Phase Series RLC Load7/LConn1
  Distributed Parameters Line12/RConn1 -- Distributed Parameters Line21/LConn1
  Distributed Parameters Line12/RConn2 -- Distributed Parameters Line21/LConn2
  Distributed Parameters Line21/RConn3 -- Three-Phase Series RLC Load6/LConn3
  Three-Phase Series RLC Load5/LConn3 -- Distributed Parameters Line7/RConn3 -- Three-Phase Series RLC Branch3/LConn3
  Three-Phase Transformer Inductance Matrix Type (Two Windings)2/LConn3 -- Three-Phase V-I Measurement/RConn3
  Three-Phase Transformer Inductance Matrix Type (Two Windings)2/LConn2 -- Three-Phase V-I Measurement/RConn2
  Three-Phase V-I Measurement8/LConn2 -- Three-Phase V-I Measurement10/LConn2 -- Three-Phase V-I Measurement11/LConn2 -- Three-Phase V-I Measurement4/RConn2
  Three-Phase Series RLC Load/LConn3 -- Three-Phase Series RLC Branch1/RConn3
  Distributed Parameters Line17/RConn1 -- Three-Phase Series RLC Load10/LConn1
  Three-Phase Series RLC Load9/LConn1 -- Distributed Parameters Line15/RConn1
  Three-Phase Series RLC Load4/LConn3 -- Distributed Parameters Line4/RConn3
  Three-Phase Series RLC Load4/LConn2 -- Distributed Parameters Line4/RConn2
  Three-Phase Transformer Inductance Matrix Type (Two Windings)2/LConn1 -- Three-Phase V-I Measurement/RConn1
  Three-Phase V-I Measurement7/RConn3 -- Distributed Parameters Line4/LConn3
  Three-Phase Series RLC Load10/LConn2 -- Distributed Parameters Line17/RConn2
  Three-Phase Transformer Inductance Matrix Type (Two Windings)1/LConn3 -- Three-Phase V-I Measurement6/RConn3
  Three-Phase Series RLC Load4/LConn1 -- Distributed Parameters Line4/RConn1
  Distributed Parameters Line21/RConn1 -- Three-Phase Series RLC Load6/LConn1
